simulink model "ODE_Hand_Model_v08_IPC"  (Simulink 7.5)
settings: Solver=ode1  StartTime=0.0  StopTime=inf  FixedStep=0.0315/(3*12)  RelTol=1e-3
values from neighbouring files (symbols this model uses):
  K_Conn = eye(4)*k_conn    [Set_Parameters.m]
  K_D = 30    [Set_Parameters.m]
  K_Or = eye(3)*k_Or    [Set_Parameters.m]
  K_Ot = eye(3)*k_Ot    [Set_Parameters.m]
  K_P = 350    [Set_Parameters.m]
  l_des = [l1_des; l2_des; l3_des; l4_des]    [Set_Parameters.m]
  R_O_Desired = R_O(x_i(qd_initial_touch))    [Set_Parameters.m]
undefined symbols (not defined in the file or in its folder): skewdec, x_desired
libraries: dspmtrx3 x30, simulink x1
settings Model: Creator=nihil  LastModifiedBy=konstantinos

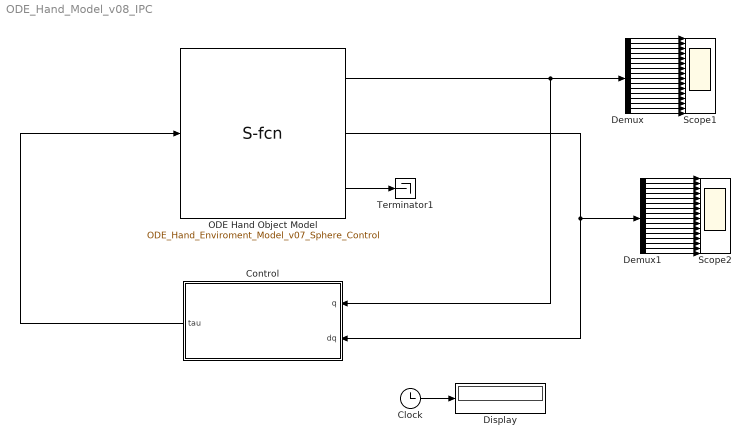
== system ODE_Hand_Model_v08_IPC ==
  Clock : Clock
      settings: Decimation=10
  Control : Subsystem
  Demux : Demux  Outputs=16
  Demux1 : Demux  Outputs=16
  Display : Display
  ODE Hand Object Model : S-Function  FunctionName=ODE_Hand_Enviroment_Model_v07_Sphere_Control  EnableBusSupport=off
  Scope1 : Scope  NumInputPorts=16
      settings: YMin=-5~-5~-5~-5~-5~-5~-5~-5~-5~-5~-5~-5~-5~-5~-5~-5  YMax=5~5~5~5~5~5~5~5~5~5~5~5~5~5~5~5
  Scope2 : Scope  NumInputPorts=16
      settings: YMin=-5~-5~-5~-5~-5~-5~-5~-5~-5~-5~-5~-5~-5~-5~-5~-5  YMax=5~5~5~5~5~5~5~5~5~5~5~5~5~5~5~5
  Terminator1 : Terminator
  wires:
  Clock/1 -> Display/1
  ODE Hand Object Model/3 -> Terminator1/1
  Control/1(tau) -> ODE Hand Object Model/1
  ODE Hand Object Model/1 -> Control/1(q), Demux/1
  ODE Hand Object Model/2 -> Control/2(dq), Demux1/1
  Demux/1 -> Scope1/1
  Demux/2 -> Scope1/2
  Demux/3 -> Scope1/3
  Demux/4 -> Scope1/4
  Demux/5 -> Scope1/5
  Demux/6 -> Scope1/6
  Demux/7 -> Scope1/7
  Demux/8 -> Scope1/8
  Demux/9 -> Scope1/9
  Demux/10 -> Scope1/10
  Demux/11 -> Scope1/11
  Demux/12 -> Scope1/12
  Demux/13 -> Scope1/13
  Demux/14 -> Scope1/14
  Demux/15 -> Scope1/15
  Demux/16 -> Scope1/16
  Demux1/1 -> Scope2/1
  Demux1/2 -> Scope2/2
  Demux1/3 -> Scope2/3
  Demux1/4 -> Scope2/4
  Demux1/5 -> Scope2/5
  Demux1/6 -> Scope2/6
  Demux1/7 -> Scope2/7
  Demux1/8 -> Scope2/8
  Demux1/9 -> Scope2/9
  Demux1/10 -> Scope2/10
  Demux1/11 -> Scope2/11
  Demux1/12 -> Scope2/12
  Demux1/13 -> Scope2/13
  Demux1/14 -> Scope2/14
  Demux1/15 -> Scope2/15
  Demux1/16 -> Scope2/16

== system ODE_Hand_Model_v08_IPC/Control ==
  q : Inport  OutDataType=fixdt(1, 16)  OutScaling=2^0
  dq : Inport  Port=2  OutDataType=fixdt(1, 16)  OutScaling=2^0
  IPC : Subsystem
  Keyboard_Guide_Touch : Subsystem
  Manual Switch : simulink/Signal Routing/Manual Switch  SystemSampleTime=-1  sw=0  action=0  varsize=off
  tau : Outport  OutDataType=fixdt(1, 16)  OutScaling=2^0
  wires:
  q/1 -> IPC/1(q), Keyboard_Guide_Touch/1(q)
  dq/1 -> Keyboard_Guide_Touch/2(dq), IPC/2(dq)
  IPC/1(tau) -> Manual Switch/1
  Keyboard_Guide_Touch/1(Out1) -> Manual Switch/2
  Manual Switch/1 -> tau/1

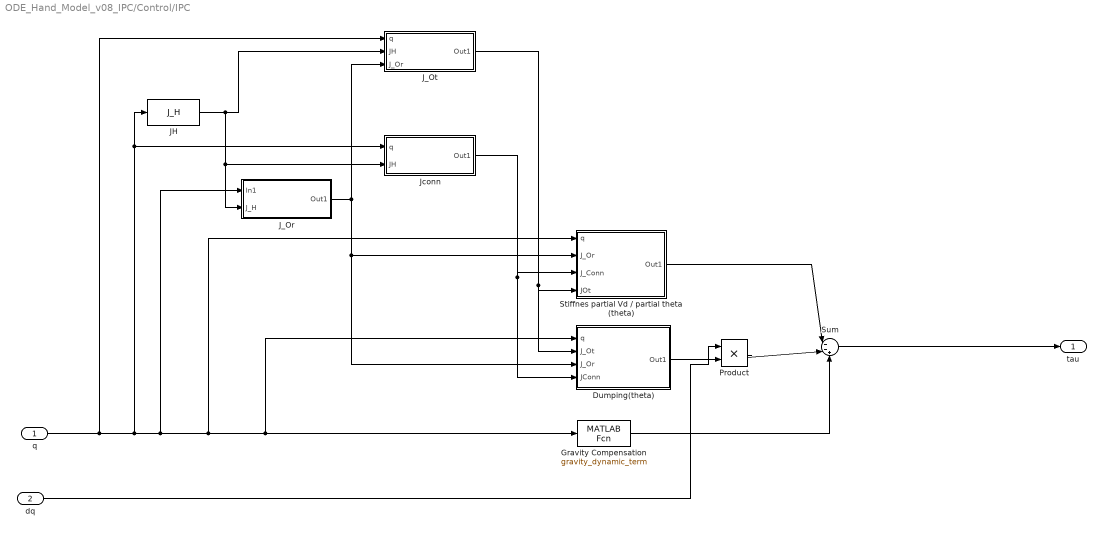
== system ODE_Hand_Model_v08_IPC/Control/IPC ==
  q : Inport  OutDataType=fixdt(1, 16)  OutScaling=2^0
  dq : Inport  Port=2  OutDataType=fixdt(1, 16)  OutScaling=2^0
  Dumping(theta) : Subsystem
  Gravity Compensation : MATLABFcn  MATLABFcn=gravity_dynamic_term  Output1D=off
  JH : MATLABFcn  MATLABFcn=J_H  Output1D=off
  J_Or : Subsystem
  J_Ot : Subsystem
  Jconn : Subsystem
  Product : Product  OutDataType=fixdt(1, 16)  OutScaling=2^0  RndMeth=Zero
  Stiffnes partial Vd / partial theta (theta) : Subsystem
  Sum : Sum  Inputs=|--+  OutDataType=fixdt(1, 16)  OutScaling=2^0
  tau : Outport  OutDataType=fixdt(1, 16)  OutScaling=2^0
  wires:
  q/1 -> Stiffnes partial Vd / partial theta (theta)/1(q), Gravity Compensation/1, Dumping(theta)/1(q), J_Or/1(In1), JH/1, Jconn/1(q), J_Ot/1(q)
  Sum/1 -> tau/1
  Gravity Compensation/1 -> Sum/3
  dq/1 -> Product/2
  Dumping(theta)/1(Out1) -> Product/1
  Product/1 -> Sum/2
  Stiffnes partial Vd / partial theta (theta)/1(Out1) -> Sum/1
  JH/1 -> J_Or/2(J_H), Jconn/2(JH), J_Ot/2(JH)
  J_Or/1(Out1) -> Dumping(theta)/3(J_Or), Stiffnes partial Vd / partial theta (theta)/2(J_Or), J_Ot/3(J_Or)
  Jconn/1(Out1) -> Dumping(theta)/4(JConn), Stiffnes partial Vd / partial theta (theta)/3(J_Conn)
  J_Ot/1(Out1) -> Stiffnes partial Vd / partial theta (theta)/4(JOt), Dumping(theta)/2(J_Ot)

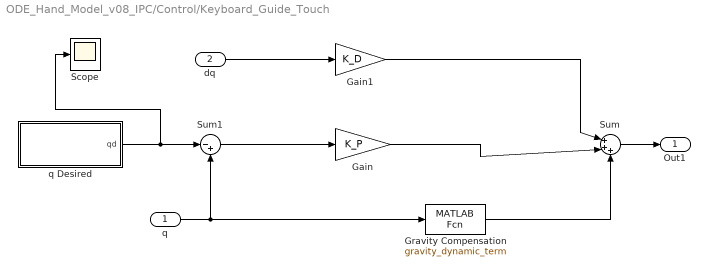
== system ODE_Hand_Model_v08_IPC/Control/Keyboard_Guide_Touch ==
  q : Inport  OutDataType=fixdt(1, 16)  OutScaling=2^0
  dq : Inport  Port=2  OutDataType=fixdt(1, 16)  OutScaling=2^0
  Gain : Gain  Gain=K_P  ParameterDataType=fixdt(1, 16)  ParameterScaling=2^0  OutDataType=fixdt(1, 16)  OutScaling=2^0
  Gain1 : Gain  Gain=K_D  ParameterDataType=fixdt(1, 16)  ParameterScaling=2^0  OutDataType=fixdt(1, 16)  OutScaling=2^0
  Gravity Compensation : MATLABFcn  MATLABFcn=gravity_dynamic_term
  Scope : Scope
      settings: SaveName=ScopeData2
  Sum : Sum  Inputs=|+++  OutDataType=fixdt(1, 16)  OutScaling=2^0
  Sum1 : Sum  Inputs=|-+  OutDataType=fixdt(1, 16)  OutScaling=2^0
  q Desired : Subsystem
  Out1 : Outport  OutDataType=fixdt(1, 16)  OutScaling=2^0
  wires:
  q/1 -> Gravity Compensation/1, Sum1/2
  Sum/1 -> Out1/1
  Sum1/1 -> Gain/1
  dq/1 -> Gain1/1
  Gain1/1 -> Sum/1
  Gain/1 -> Sum/2
  q Desired/1(qd) -> Sum1/1, Scope/1
  Gravity Compensation/1 -> Sum/3

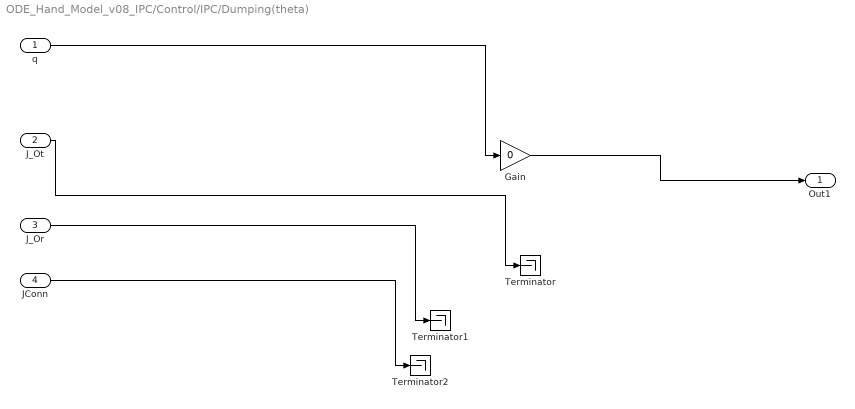
== system ODE_Hand_Model_v08_IPC/Control/IPC/Dumping(theta) ==
  q : Inport  OutDataType=fixdt(1, 16)  OutScaling=2^0
  J_Ot : Inport  Port=2  OutDataType=fixdt(1, 16)  OutScaling=2^0
  J_Or : Inport  Port=3  OutDataType=fixdt(1, 16)  OutScaling=2^0
  JConn : Inport  Port=4  OutDataType=fixdt(1, 16)  OutScaling=2^0
  Gain : Gain  Gain=0  ParameterDataType=fixdt(1, 16)  ParameterScaling=2^0  OutDataType=fixdt(1, 16)  OutScaling=2^0
  Terminator : Terminator
  Terminator1 : Terminator
  Terminator2 : Terminator
  Out1 : Outport  OutDataType=fixdt(1, 16)  OutScaling=2^0
  wires:
  q/1 -> Gain/1
  J_Ot/1 -> Terminator/1
  J_Or/1 -> Terminator1/1
  JConn/1 -> Terminator2/1
  Gain/1 -> Out1/1

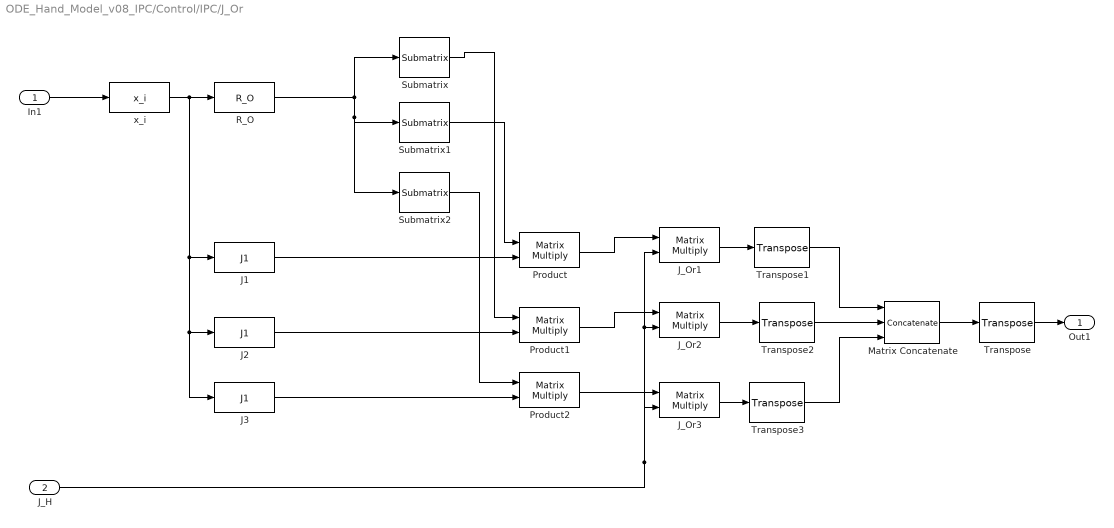
== system ODE_Hand_Model_v08_IPC/Control/IPC/J_Or ==
  In1 : Inport  OutDataType=fixdt(1, 16)  OutScaling=2^0
  J_H : Inport  Port=2  OutDataType=fixdt(1, 16)  OutScaling=2^0
  J1 : MATLABFcn  MATLABFcn=J1  Output1D=off
  J2 : MATLABFcn  MATLABFcn=J1  Output1D=off
  J3 : MATLABFcn  MATLABFcn=J1  Output1D=off
  J_Or1 : Product  Multiplication=Matrix(*)  OutDataType=fixdt(1, 16)  OutScaling=2^0  RndMeth=Zero
  J_Or2 : Product  Multiplication=Matrix(*)  OutDataType=fixdt(1, 16)  OutScaling=2^0  RndMeth=Zero
  J_Or3 : Product  Multiplication=Matrix(*)  OutDataType=fixdt(1, 16)  OutScaling=2^0  RndMeth=Zero
  Matrix Concatenate : Concatenate  NumInputs=3  Mode=Multidimensional array  ConcatenateDimension=2
  Product : Product  Multiplication=Matrix(*)  OutDataType=fixdt(1, 16)  OutScaling=2^0  RndMeth=Zero
  Product1 : Product  Multiplication=Matrix(*)  OutDataType=fixdt(1, 16)  OutScaling=2^0  RndMeth=Zero
  Product2 : Product  Multiplication=Matrix(*)  OutDataType=fixdt(1, 16)  OutScaling=2^0  RndMeth=Zero
  R_O : MATLABFcn  MATLABFcn=R_O  OutputSignalType=real  Output1D=off
  Submatrix : dspmtrx3/Submatrix  RowSpan=One row  RowStartMode=First  RowStartIndex=1  RowEndMode=Last  RowEndIndex=1  ColSpan=All columns  ColStartMode=First  ColStartIndex=1  ColEndMode=Last  ColEndIndex=1
  Submatrix1 : dspmtrx3/Submatrix  RowSpan=One row  RowStartMode=Index  RowStartIndex=2  RowEndMode=Last  RowEndIndex=1  ColSpan=All columns  ColStartMode=First  ColStartIndex=1  ColEndMode=Last  ColEndIndex=1
  Submatrix2 : dspmtrx3/Submatrix  RowSpan=One row  RowStartMode=Index  RowStartIndex=3  RowEndMode=Last  RowEndIndex=1  ColSpan=All columns  ColStartMode=First  ColStartIndex=1  ColEndMode=Last  ColEndIndex=1
  Transpose{,1..3} (4 alike) : dspmtrx3/Transpose  SystemSampleTime=-1  Hermitian=off  overflowFlag=off
  x_i : MATLABFcn  MATLABFcn=x_i  Output1D=off
  Out1 : Outport  OutDataType=fixdt(1, 16)  OutScaling=2^0
  wires:
  x_i/1 -> R_O/1, J1/1, J2/1, J3/1
  R_O/1 -> Submatrix/1, Submatrix1/1, Submatrix2/1
  In1/1 -> x_i/1
  Submatrix1/1 -> Product/1
  J1/1 -> Product/2
  Submatrix/1 -> Product1/1
  Submatrix2/1 -> Product2/1
  J2/1 -> Product1/2
  J3/1 -> Product2/2
  Product/1 -> J_Or1/1
  Product1/1 -> J_Or2/1
  Product2/1 -> J_Or3/1
  J_H/1 -> J_Or3/2, J_Or2/2, J_Or1/2
  Matrix Concatenate/1 -> Transpose/1
  Transpose/1 -> Out1/1
  J_Or1/1 -> Transpose1/1
  J_Or2/1 -> Transpose2/1
  J_Or3/1 -> Transpose3/1
  Transpose2/1 -> Matrix Concatenate/2
  Transpose1/1 -> Matrix Concatenate/1
  Transpose3/1 -> Matrix Concatenate/3

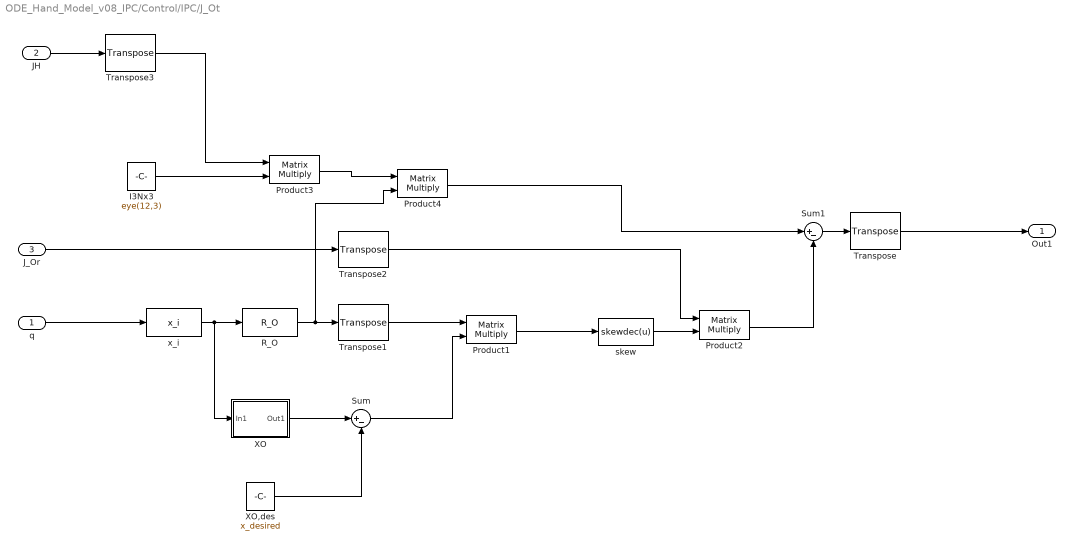
== system ODE_Hand_Model_v08_IPC/Control/IPC/J_Ot ==
  q : Inport  OutDataType=fixdt(1, 16)  OutScaling=2^0
  JH : Inport  Port=2  OutDataType=fixdt(1, 16)  OutScaling=2^0
  J_Or : Inport  Port=3  OutDataType=fixdt(1, 16)  OutScaling=2^0
  I3Nx3 : Constant  Value=eye(12,3)  OutDataType=fixdt(1, 16)  OutScaling=2^0
  Product{1..4} (4 alike) : Product  Multiplication=Matrix(*)  OutDataType=fixdt(1, 16)  OutScaling=2^0  RndMeth=Zero
  R_O : MATLABFcn  MATLABFcn=R_O  OutputSignalType=real  Output1D=off
  Sum : Sum  Inputs=|+-  OutDataType=fixdt(1, 16)  OutScaling=2^0
  Sum1 : Sum  Inputs=|+-  OutDataType=fixdt(1, 16)  OutScaling=2^0
  Transpose{,1..3} (4 alike) : dspmtrx3/Transpose  SystemSampleTime=-1  Hermitian=off  overflowFlag=off
  XO : Subsystem
  XO,des : Constant  Value=x_desired  OutDataType=fixdt(1, 16)  OutScaling=2^0
  skew : MATLABFcn  MATLABFcn=skewdec(u)  Output1D=off
  x_i : MATLABFcn  MATLABFcn=x_i  Output1D=off
  Out1 : Outport  OutDataType=fixdt(1, 16)  OutScaling=2^0
  wires:
  q/1 -> x_i/1
  x_i/1 -> R_O/1, XO/1(In1)
  R_O/1 -> Transpose1/1, Product4/2
  XO/1(Out1) -> Sum/1
  XO,des/1 -> Sum/2
  Sum/1 -> Product1/2
  Transpose1/1 -> Product1/1
  Product1/1 -> skew/1
  skew/1 -> Product2/2
  J_Or/1 -> Transpose2/1
  Transpose2/1 -> Product2/1
  Product2/1 -> Sum1/2
  JH/1 -> Transpose3/1
  Product4/1 -> Sum1/1
  I3Nx3/1 -> Product3/2
  Transpose3/1 -> Product3/1
  Product3/1 -> Product4/1
  Sum1/1 -> Transpose/1
  Transpose/1 -> Out1/1

== system ODE_Hand_Model_v08_IPC/Control/IPC/Jconn ==
  q : Inport  OutDataType=fixdt(1, 16)  OutScaling=2^0
  JH : Inport  Port=2  OutDataType=fixdt(1, 16)  OutScaling=2^0
  Product2 : Product  Multiplication=Matrix(*)  OutDataType=fixdt(1, 16)  OutScaling=2^0  RndMeth=Zero
  Transpose : dspmtrx3/Transpose  SystemSampleTime=-1  Hermitian=off  overflowFlag=off
  Transpose1 : dspmtrx3/Transpose  SystemSampleTime=-1  Hermitian=off  overflowFlag=off
  partial_x : MATLABFcn  MATLABFcn=partial_x  OutputSignalType=real  Output1D=off
  x_i : MATLABFcn  MATLABFcn=x_i  Output1D=off
  Out1 : Outport  OutDataType=fixdt(1, 16)  OutScaling=2^0
  wires:
  x_i/1 -> partial_x/1
  Transpose/1 -> Product2/1
  partial_x/1 -> Product2/2
  JH/1 -> Transpose/1
  q/1 -> x_i/1
  Product2/1 -> Transpose1/1
  Transpose1/1 -> Out1/1

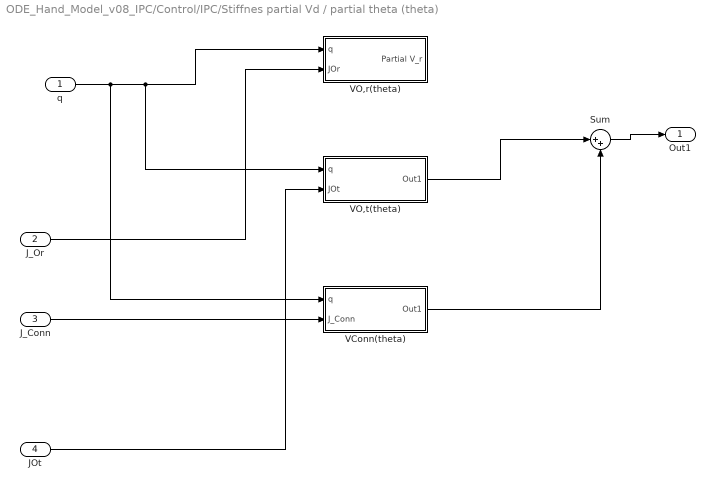
== system ODE_Hand_Model_v08_IPC/Control/IPC/Stiffnes partial Vd / partial theta (theta) ==
  q : Inport  OutDataType=fixdt(1, 16)  OutScaling=2^0
  J_Or : Inport  Port=2  OutDataType=fixdt(1, 16)  OutScaling=2^0
  J_Conn : Inport  Port=3  OutDataType=fixdt(1, 16)  OutScaling=2^0
  JOt : Inport  Port=4  OutDataType=fixdt(1, 16)  OutScaling=2^0
  Sum : Sum  Inputs=|++  OutDataType=fixdt(1, 16)  OutScaling=2^0
  VConn(theta) : Subsystem
  VO,r(theta) : Subsystem
  VO,t(theta) : Subsystem
  Out1 : Outport  OutDataType=fixdt(1, 16)  OutScaling=2^0
  wires:
  q/1 -> VO,r(theta)/1(q), VO,t(theta)/1(q), VConn(theta)/1(q)
  Sum/1 -> Out1/1
  J_Conn/1 -> VConn(theta)/2(J_Conn)
  J_Or/1 -> VO,r(theta)/2(JOr)
  JOt/1 -> VO,t(theta)/2(JOt)
  VO,t(theta)/1(Out1) -> Sum/1
  VConn(theta)/1(Out1) -> Sum/2

== system ODE_Hand_Model_v08_IPC/Control/Keyboard_Guide_Touch/q Desired ==
  Demux1 : Demux  Outputs=16
  Discrete State-Space : DiscreteStateSpace  A=eye(16)  B=eye(16)  C=eye(16)  D=zeros(16)  X0=zeros(1,16)  SampleTime=-1
  Level-2 M-file S-Function : M-S-Function  FunctionName=sfun_keyboard_input_v1_2
  Product : Product  OutDataType=fixdt(1, 16)  OutScaling=2^0  RndMeth=Zero
  Scope2 : Scope  NumInputPorts=16
      settings: YMin=-5~-5~-5~-5~-5~-5~-5~-5~-5~-5~-5~-5~-5~-5~-5~-5  YMax=5~5~5~5~5~5~5~5~5~5~5~5~5~5~5~5  SaveName=ScopeData3
  q_d : MATLABFcn  MATLABFcn=q_d
  qd : Outport  OutDataType=fixdt(1, 16)  OutScaling=2^0
  wires:
  Level-2 M-file S-Function/2 -> Product/2
  Level-2 M-file S-Function/1 -> Product/1
  Discrete State-Space/1 -> qd/1, Demux1/1
  Product/1 -> q_d/1
  Demux1/1 -> Scope2/1
  Demux1/2 -> Scope2/2
  Demux1/3 -> Scope2/3
  Demux1/4 -> Scope2/4
  Demux1/5 -> Scope2/5
  Demux1/6 -> Scope2/6
  Demux1/7 -> Scope2/7
  Demux1/8 -> Scope2/8
  Demux1/9 -> Scope2/9
  Demux1/10 -> Scope2/10
  Demux1/11 -> Scope2/11
  Demux1/12 -> Scope2/12
  Demux1/13 -> Scope2/13
  Demux1/14 -> Scope2/14
  Demux1/15 -> Scope2/15
  Demux1/16 -> Scope2/16
  q_d/1 -> Discrete State-Space/1

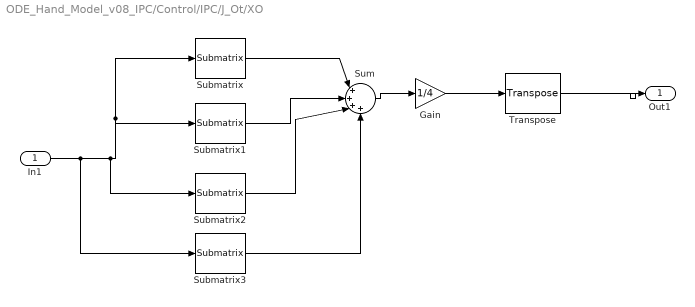
== system ODE_Hand_Model_v08_IPC/Control/IPC/J_Ot/XO ==
  In1 : Inport  OutDataType=fixdt(1, 16)  OutScaling=2^0
  Gain : Gain  Gain=1/4  ParameterDataType=fixdt(1, 16)  ParameterScaling=2^0  OutDataType=fixdt(1, 16)  OutScaling=2^0
  Submatrix : dspmtrx3/Submatrix  RowSpan=One row  RowStartMode=First  RowStartIndex=1  RowEndMode=Last  RowEndIndex=1  ColSpan=All columns  ColStartMode=First  ColStartIndex=1  ColEndMode=Last  ColEndIndex=1
  Submatrix1 : dspmtrx3/Submatrix  RowSpan=One row  RowStartMode=Index  RowStartIndex=1  RowEndMode=Last  RowEndIndex=1  ColSpan=All columns  ColStartMode=First  ColStartIndex=1  ColEndMode=Last  ColEndIndex=1
  Submatrix2 : dspmtrx3/Submatrix  RowSpan=One row  RowStartMode=Index  RowStartIndex=3  RowEndMode=Last  RowEndIndex=1  ColSpan=All columns  ColStartMode=First  ColStartIndex=1  ColEndMode=Last  ColEndIndex=1
  Submatrix3 : dspmtrx3/Submatrix  RowSpan=One row  RowStartMode=Last  RowStartIndex=1  RowEndMode=Last  RowEndIndex=1  ColSpan=All columns  ColStartMode=First  ColStartIndex=1  ColEndMode=Last  ColEndIndex=1
  Sum : Sum  Inputs=|++++  OutDataType=fixdt(1, 16)  OutScaling=2^0
  Transpose : dspmtrx3/Transpose  SystemSampleTime=-1  Hermitian=off  overflowFlag=off
  Out1 : Outport  OutDataType=fixdt(1, 16)  OutScaling=2^0
  wires:
  In1/1 -> Submatrix/1, Submatrix1/1, Submatrix2/1, Submatrix3/1
  Sum/1 -> Gain/1
  Submatrix/1 -> Sum/1
  Submatrix1/1 -> Sum/2
  Submatrix2/1 -> Sum/3
  Submatrix3/1 -> Sum/4
  Gain/1 -> Transpose/1
  Transpose/1 -> Out1/1

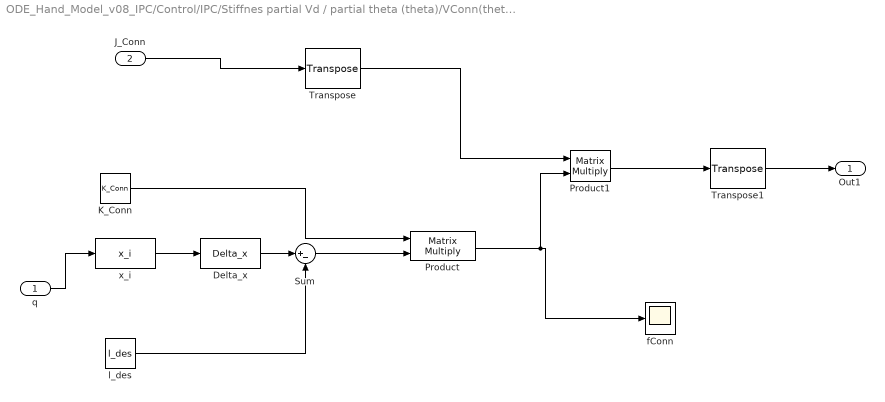
== system ODE_Hand_Model_v08_IPC/Control/IPC/Stiffnes partial Vd / partial theta (theta)/VConn(theta) ==
  q : Inport  OutDataType=fixdt(1, 16)  OutScaling=2^0
  J_Conn : Inport  Port=2  OutDataType=fixdt(1, 16)  OutScaling=2^0
  Delta_x : MATLABFcn  MATLABFcn=Delta_x  Output1D=off
  K_Conn : Constant  Value=K_Conn  OutDataType=fixdt(1, 16)  OutScaling=2^0
  Product : Product  Multiplication=Matrix(*)  OutDataType=fixdt(1, 16)  OutScaling=2^0  RndMeth=Zero
  Product1 : Product  Multiplication=Matrix(*)  OutDataType=fixdt(1, 16)  OutScaling=2^0  RndMeth=Zero
  Sum : Sum  Inputs=|+-  OutDataType=fixdt(1, 16)  OutScaling=2^0
  Transpose : dspmtrx3/Transpose  SystemSampleTime=-1  Hermitian=off  overflowFlag=off
  Transpose1 : dspmtrx3/Transpose  SystemSampleTime=-1  Hermitian=off  overflowFlag=off
  fConn : Scope
      settings: SaveName=ScopeData5
  l_des : Constant  Value=l_des  OutDataType=fixdt(1, 16)  OutScaling=2^0
  x_i : MATLABFcn  MATLABFcn=x_i  Output1D=off
  Out1 : Outport  OutDataType=fixdt(1, 16)  OutScaling=2^0
  wires:
  q/1 -> x_i/1
  x_i/1 -> Delta_x/1
  Delta_x/1 -> Sum/1
  l_des/1 -> Sum/2
  Sum/1 -> Product/2
  Product/1 -> fConn/1, Product1/2
  K_Conn/1 -> Product/1
  J_Conn/1 -> Transpose/1
  Transpose/1 -> Product1/1
  Product1/1 -> Transpose1/1
  Transpose1/1 -> Out1/1

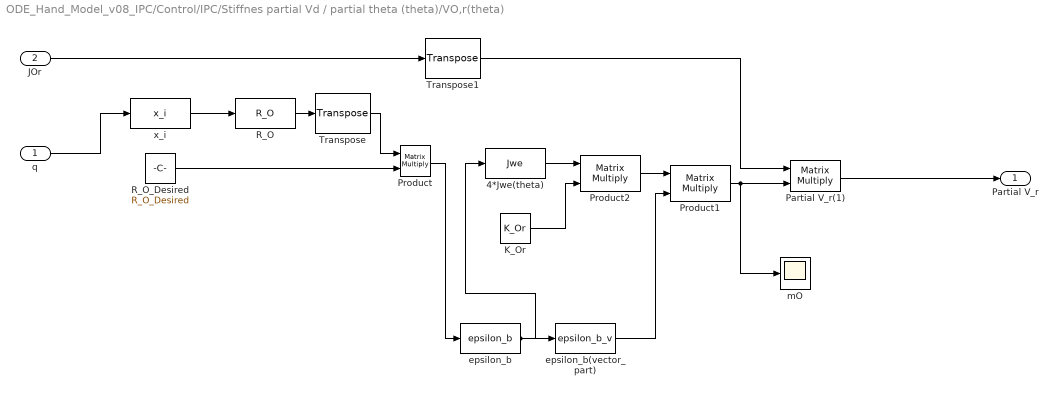
== system ODE_Hand_Model_v08_IPC/Control/IPC/Stiffnes partial Vd / partial theta (theta)/VO,r(theta) ==
  q : Inport  OutDataType=fixdt(1, 16)  OutScaling=2^0
  JOr : Inport  Port=2  OutDataType=fixdt(1, 16)  OutScaling=2^0
  4*Jwe(theta) : MATLABFcn  MATLABFcn=Jwe  Output1D=off
  K_Or : Constant  Value=K_Or  OutDataType=fixdt(1, 16)  OutScaling=2^0
  Partial V_r(1) : Product  Multiplication=Matrix(*)  OutDataType=fixdt(1, 16)  OutScaling=2^0  RndMeth=Zero
  Product : Product  Multiplication=Matrix(*)  OutDataType=fixdt(1, 16)  OutScaling=2^0  RndMeth=Zero
  Product1 : Product  Multiplication=Matrix(*)  OutDataType=fixdt(1, 16)  OutScaling=2^0  RndMeth=Zero
  Product2 : Product  Multiplication=Matrix(*)  OutDataType=fixdt(1, 16)  OutScaling=2^0  RndMeth=Zero
  R_O : MATLABFcn  MATLABFcn=R_O  OutputSignalType=real  Output1D=off
  R_O_Desired : Constant  Value=R_O_Desired  OutDataType=fixdt(1, 16)  OutScaling=2^0
  Transpose : dspmtrx3/Transpose  SystemSampleTime=-1  Hermitian=off  overflowFlag=off
  Transpose1 : dspmtrx3/Transpose  SystemSampleTime=-1  Hermitian=off  overflowFlag=off
  epsilon_b : MATLABFcn  MATLABFcn=epsilon_b  Output1D=off
  epsilon_b(vector_part) : MATLABFcn  MATLABFcn=epsilon_b_v  Output1D=off
  mO : Scope
      settings: SaveName=ScopeData4
  x_i : MATLABFcn  MATLABFcn=x_i  Output1D=off
  Partial V_r : Outport  OutDataType=fixdt(1, 16)  OutScaling=2^0
  wires:
  q/1 -> x_i/1
  x_i/1 -> R_O/1
  Product/1 -> epsilon_b/1
  Product1/1 -> mO/1, Partial V_r(1)/2
  4*Jwe(theta)/1 -> Product2/1
  K_Or/1 -> Product2/2
  Product2/1 -> Product1/1
  epsilon_b/1 -> 4*Jwe(theta)/1, epsilon_b(vector_part)/1
  epsilon_b(vector_part)/1 -> Product1/2
  Transpose1/1 -> Partial V_r(1)/1
  Partial V_r(1)/1 -> Partial V_r/1
  R_O_Desired/1 -> Product/2
  R_O/1 -> Transpose/1
  Transpose/1 -> Product/1
  JOr/1 -> Transpose1/1

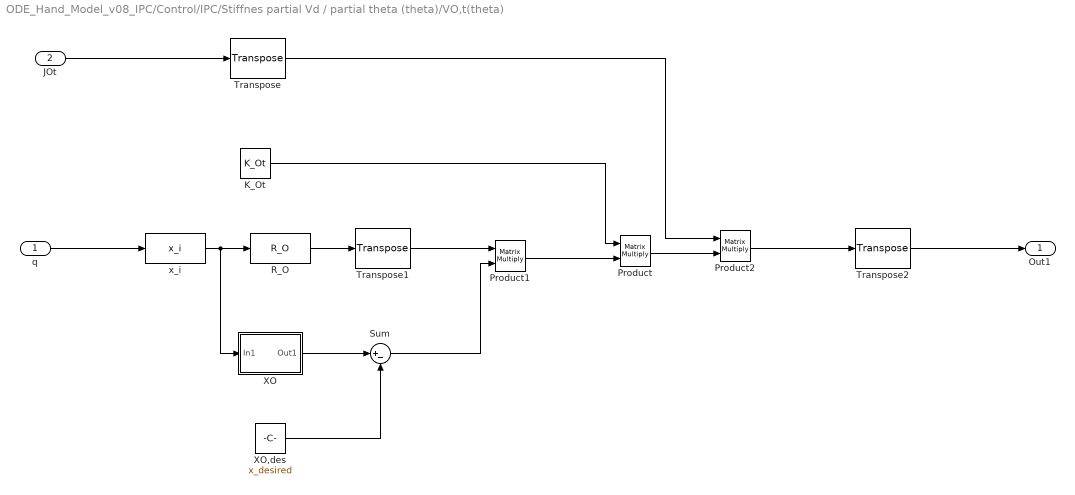
== system ODE_Hand_Model_v08_IPC/Control/IPC/Stiffnes partial Vd / partial theta (theta)/VO,t(theta) ==
  q : Inport  OutDataType=fixdt(1, 16)  OutScaling=2^0
  JOt : Inport  Port=2  OutDataType=fixdt(1, 16)  OutScaling=2^0
  K_Ot : Constant  Value=K_Ot  OutDataType=fixdt(1, 16)  OutScaling=2^0
  Product : Product  Multiplication=Matrix(*)  OutDataType=fixdt(1, 16)  OutScaling=2^0  RndMeth=Zero
  Product1 : Product  Multiplication=Matrix(*)  OutDataType=fixdt(1, 16)  OutScaling=2^0  RndMeth=Zero
  Product2 : Product  Multiplication=Matrix(*)  OutDataType=fixdt(1, 16)  OutScaling=2^0  RndMeth=Zero
  R_O : MATLABFcn  MATLABFcn=R_O  OutputSignalType=real  Output1D=off
  Sum : Sum  Inputs=|+-  OutDataType=fixdt(1, 16)  OutScaling=2^0
  Transpose : dspmtrx3/Transpose  SystemSampleTime=-1  Hermitian=off  overflowFlag=off
  Transpose1 : dspmtrx3/Transpose  SystemSampleTime=-1  Hermitian=off  overflowFlag=off
  Transpose2 : dspmtrx3/Transpose  SystemSampleTime=-1  Hermitian=off  overflowFlag=off
  XO : Subsystem
  XO,des : Constant  Value=x_desired  OutDataType=fixdt(1, 16)  OutScaling=2^0
  x_i : MATLABFcn  MATLABFcn=x_i  Output1D=off
  Out1 : Outport  OutDataType=fixdt(1, 16)  OutScaling=2^0
  wires:
  q/1 -> x_i/1
  JOt/1 -> Transpose/1
  x_i/1 -> R_O/1, XO/1(In1)
  R_O/1 -> Transpose1/1
  XO/1(Out1) -> Sum/1
  XO,des/1 -> Sum/2
  Sum/1 -> Product1/2
  Transpose1/1 -> Product1/1
  Product1/1 -> Product/2
  K_Ot/1 -> Product/1
  Product/1 -> Product2/2
  Transpose/1 -> Product2/1
  Product2/1 -> Transpose2/1
  Transpose2/1 -> Out1/1

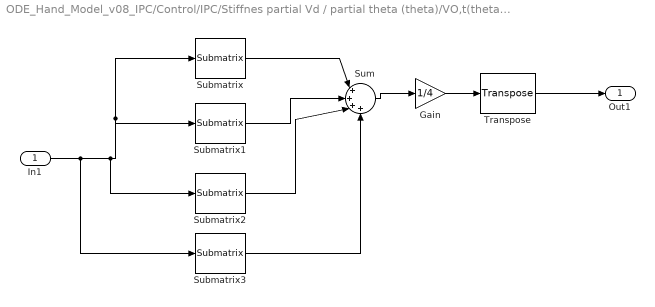
== system ODE_Hand_Model_v08_IPC/Control/IPC/Stiffnes partial Vd / partial theta (theta)/VO,t(theta)/XO ==
  In1 : Inport  OutDataType=fixdt(1, 16)  OutScaling=2^0
  Gain : Gain  Gain=1/4  ParameterDataType=fixdt(1, 16)  ParameterScaling=2^0  OutDataType=fixdt(1, 16)  OutScaling=2^0
  Submatrix : dspmtrx3/Submatrix  RowSpan=One row  RowStartMode=First  RowStartIndex=1  RowEndMode=Last  RowEndIndex=1  ColSpan=All columns  ColStartMode=First  ColStartIndex=1  ColEndMode=Last  ColEndIndex=1
  Submatrix1 : dspmtrx3/Submatrix  RowSpan=One row  RowStartMode=Index  RowStartIndex=1  RowEndMode=Last  RowEndIndex=1  ColSpan=All columns  ColStartMode=First  ColStartIndex=1  ColEndMode=Last  ColEndIndex=1
  Submatrix2 : dspmtrx3/Submatrix  RowSpan=One row  RowStartMode=Index  RowStartIndex=3  RowEndMode=Last  RowEndIndex=1  ColSpan=All columns  ColStartMode=First  ColStartIndex=1  ColEndMode=Last  ColEndIndex=1
  Submatrix3 : dspmtrx3/Submatrix  RowSpan=One row  RowStartMode=Last  RowStartIndex=1  RowEndMode=Last  RowEndIndex=1  ColSpan=All columns  ColStartMode=First  ColStartIndex=1  ColEndMode=Last  ColEndIndex=1
  Sum : Sum  Inputs=|++++  OutDataType=fixdt(1, 16)  OutScaling=2^0
  Transpose : dspmtrx3/Transpose  SystemSampleTime=-1  Hermitian=off  overflowFlag=off
  Out1 : Outport  OutDataType=fixdt(1, 16)  OutScaling=2^0
  wires:
  In1/1 -> Submatrix/1, Submatrix1/1, Submatrix2/1, Submatrix3/1
  Sum/1 -> Gain/1
  Submatrix/1 -> Sum/1
  Submatrix1/1 -> Sum/2
  Submatrix2/1 -> Sum/3
  Submatrix3/1 -> Sum/4
  Gain/1 -> Transpose/1
  Transpose/1 -> Out1/1
